simulink model "EstudioReguladores"  (R2024b)
settings: Solver=VariableStepAuto  StartTime=0.0  StopTime=50000  RelTol=1e-3
undefined symbols (not defined in the file): n, p1, p2, p3, Vi
libraries: slpidlib x32
(part 1 of 4)
settings Model: Creator=HP  LastModifiedBy=HP

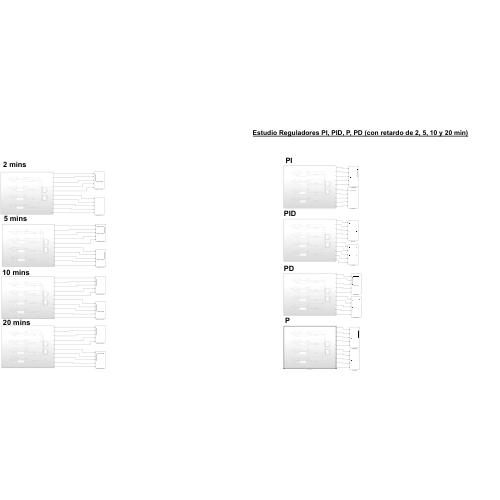
[thumbnail: Simulink's stored preview of the top-level diagram]
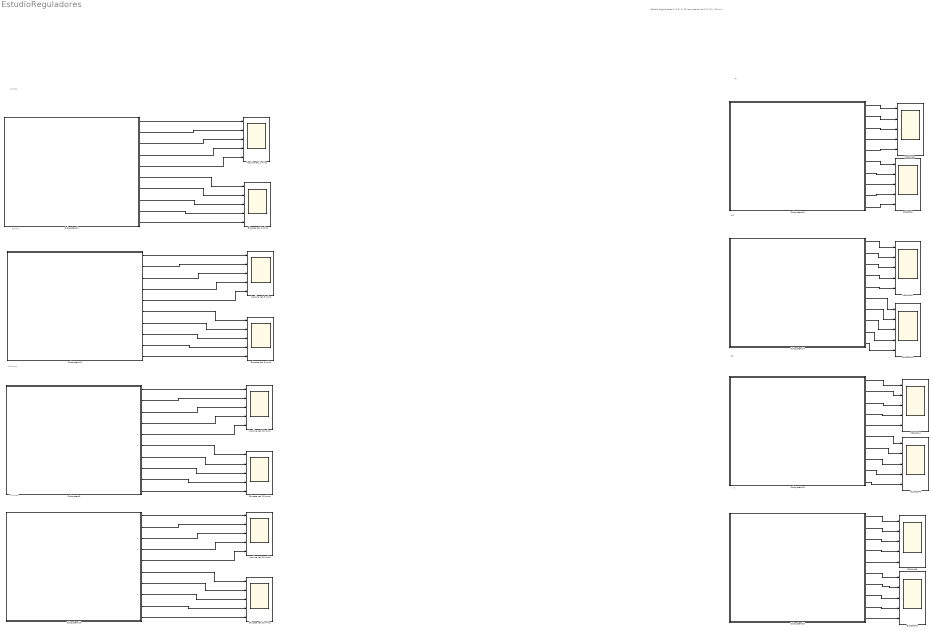
== system EstudioReguladores ==
  note: PI
  note: PID
  note: P
  note: 5 mins
  note: 2 mins
  note: Estudio Reguladores PI, PID, P, PD (con retardo de 2, 5, 10 y 20 min)
  note: 10 mins
  note: PD
  note: 20 mins
  GLUCOSA{,1..3} (4 alike) : Scope  NumInputPorts=5
  Glucosa ret. 10 mins. : Scope  NumInputPorts=5
  Glucosa ret. 2 mins : Scope  NumInputPorts=5
  Glucosa ret. 20 mins. : Scope  NumInputPorts=5
  Glucosa ret. 5 mins. : Scope  NumInputPorts=5
  INSULINA{2..5} (4 alike) : Scope  NumInputPorts=5
  Insulina ret. 10 mins. : Scope  NumInputPorts=5
  Insulina ret. 2 mins : Scope  NumInputPorts=5
  Insulina ret. 20 mins. : Scope  NumInputPorts=5
  Insulina ret. 5 mins. : Scope  NumInputPorts=5
  Subsystem10 : Subsystem
  Subsystem11 : Subsystem
  Subsystem12 : Subsystem
  Subsystem13 : Subsystem
  Subsystem14 : Subsystem
  Subsystem15 : Subsystem
  Subsystem16 : Subsystem
  Subsystem9 : Subsystem
  wires:
  Subsystem11/5(Out5) -> Insulina ret. 2 mins/5
  Subsystem16/7(Out7) -> GLUCOSA3/2
  Subsystem10/2(Out2) -> Insulina ret. 20 mins./2
  Subsystem11/3(Out3) -> Insulina ret. 2 mins/3
  Subsystem13/2(Out2) -> INSULINA2/2
  Subsystem13/10(Out10) -> GLUCOSA/5
  Subsystem10/4(Out4) -> Insulina ret. 20 mins./4
  Subsystem12/2(Out2) -> Insulina ret. 5 mins./2
  Subsystem13/1(Out1) -> INSULINA2/1
  Subsystem10/9(Out9) -> Glucosa ret. 20 mins./4
  Subsystem10/5(Out5) -> Insulina ret. 20 mins./5
  Subsystem10/1(Out1) -> Insulina ret. 20 mins./1
  Subsystem14/2(Out2) -> INSULINA3/2
  Subsystem12/4(Out4) -> Insulina ret. 5 mins./4
  Subsystem9/9(Out9) -> Glucosa ret. 10 mins./4
  Subsystem13/9(Out9) -> GLUCOSA/4
  Subsystem10/3(Out3) -> Insulina ret. 20 mins./3
  Subsystem14/7(Out7) -> GLUCOSA1/2
  Subsystem12/5(Out5) -> Insulina ret. 5 mins./5
  Subsystem12/1(Out1) -> Insulina ret. 5 mins./1
  Subsystem10/7(Out7) -> Glucosa ret. 20 mins./2
  Subsystem11/9(Out9) -> Glucosa ret. 2 mins/4
  Subsystem12/7(Out7) -> Glucosa ret. 5 mins./2
  Subsystem9/3(Out3) -> Insulina ret. 10 mins./3
  Subsystem11/1(Out1) -> Insulina ret. 2 mins/1
  Subsystem11/10(Out10) -> Glucosa ret. 2 mins/5
  Subsystem11/7(Out7) -> Glucosa ret. 2 mins/2
  Subsystem13/3(Out3) -> INSULINA2/3
  Subsystem16/6(Out6) -> GLUCOSA3/1
  Subsystem13/5(Out5) -> INSULINA2/5
  Subsystem15/8(Out8) -> GLUCOSA2/3
  Subsystem16/1(Out1) -> INSULINA5/1
  Subsystem13/4(Out4) -> INSULINA2/4
  Subsystem15/7(Out7) -> GLUCOSA2/2
  Subsystem9/5(Out5) -> Insulina ret. 10 mins./5
  Subsystem12/6(Out6) -> Glucosa ret. 5 mins./1
  Subsystem13/7(Out7) -> GLUCOSA/2
  Subsystem11/4(Out4) -> Insulina ret. 2 mins/4
  Subsystem9/10(Out10) -> Glucosa ret. 10 mins./5
  Subsystem12/9(Out9) -> Glucosa ret. 5 mins./4
  Subsystem9/1(Out1) -> Insulina ret. 10 mins./1
  Subsystem9/8(Out8) -> Glucosa ret. 10 mins./3
  Subsystem11/2(Out2) -> Insulina ret. 2 mins/2
  Subsystem9/7(Out7) -> Glucosa ret. 10 mins./2
  Subsystem13/6(Out6) -> GLUCOSA/1
  Subsystem12/10(Out10) -> Glucosa ret. 5 mins./5
  Subsystem11/6(Out6) -> Glucosa ret. 2 mins/1
  Subsystem13/8(Out8) -> GLUCOSA/3
  Subsystem9/4(Out4) -> Insulina ret. 10 mins./4
  Subsystem10/10(Out10) -> Glucosa ret. 20 mins./5
  Subsystem10/8(Out8) -> Glucosa ret. 20 mins./3
  Subsystem12/8(Out8) -> Glucosa ret. 5 mins./3
  Subsystem11/8(Out8) -> Glucosa ret. 2 mins/3
  Subsystem9/2(Out2) -> Insulina ret. 10 mins./2
  Subsystem10/6(Out6) -> Glucosa ret. 20 mins./1
  Subsystem12/3(Out3) -> Insulina ret. 5 mins./3
  Subsystem9/6(Out6) -> Glucosa ret. 10 mins./1
  Subsystem15/6(Out6) -> GLUCOSA2/1
  Subsystem14/6(Out6) -> GLUCOSA1/1
  Subsystem14/8(Out8) -> GLUCOSA1/3
  Subsystem14/9(Out9) -> GLUCOSA1/4
  Subsystem14/10(Out10) -> GLUCOSA1/5
  Subsystem14/1(Out1) -> INSULINA3/1
  Subsystem14/3(Out3) -> INSULINA3/3
  Subsystem14/4(Out4) -> INSULINA3/4
  Subsystem14/5(Out5) -> INSULINA3/5
  Subsystem15/1(Out1) -> INSULINA4/1
  Subsystem15/2(Out2) -> INSULINA4/2
  Subsystem15/3(Out3) -> INSULINA4/3
  Subsystem15/4(Out4) -> INSULINA4/4
  Subsystem15/5(Out5) -> INSULINA4/5
  Subsystem16/2(Out2) -> INSULINA5/2
  Subsystem16/3(Out3) -> INSULINA5/3
  Subsystem16/4(Out4) -> INSULINA5/4
  Subsystem16/5(Out5) -> INSULINA5/5
  Subsystem15/9(Out9) -> GLUCOSA2/4
  Subsystem15/10(Out10) -> GLUCOSA2/5
  Subsystem16/8(Out8) -> GLUCOSA3/3
  Subsystem16/9(Out9) -> GLUCOSA3/4
  Subsystem16/10(Out10) -> GLUCOSA3/5

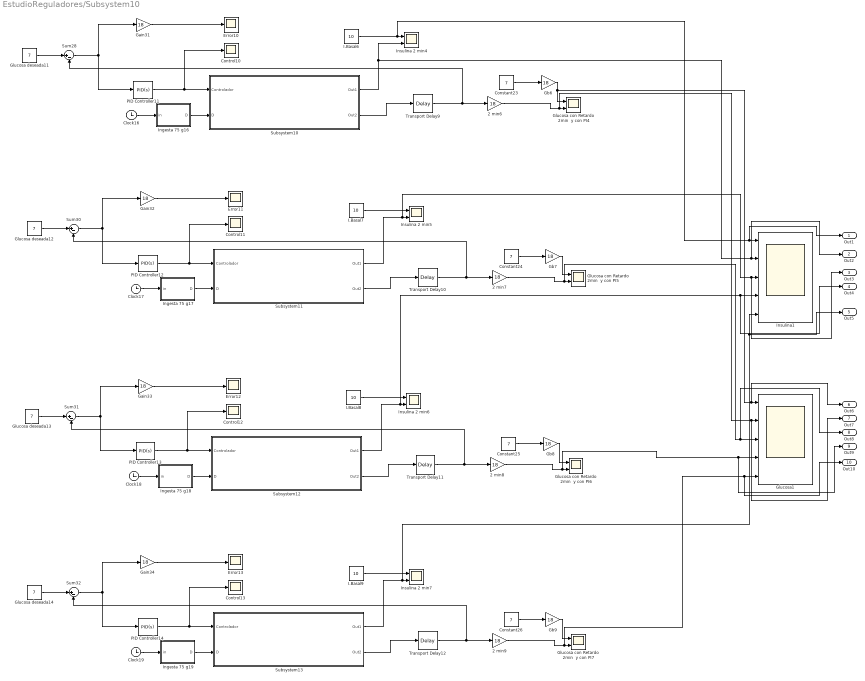
== system EstudioReguladores/Subsystem10 ==
  2 min{6..9} (4 alike) : Gain  Gain=18
  Clock{16..19} (4 alike) : Clock
  Constant{23..26} (4 alike) : Constant  Value=7
  Control{10..13} (4 alike) : Scope
  Error{10..13} (4 alike) : Scope
  Gain{31..34} (4 alike) : Gain  Gain=18
  Gb{6..9} (4 alike) : Gain  Gain=18
  Glucosa con Retardo 2min  y con PI{4..7} (4 alike) : Scope  NumInputPorts=2
  Glucosa deseada{11..14} (4 alike) : Constant  Value=7
  Glucosa1 : Scope  NumInputPorts=5
  I.Basal{6..9} (4 alike) : Constant  Value=10
  Ingesta 75 g16 : MATLAB Function  TreatAsAtomicUnit=on
  Ingesta 75 g17 : MATLAB Function  TreatAsAtomicUnit=on
  Ingesta 75 g18 : MATLAB Function  TreatAsAtomicUnit=on
  Ingesta 75 g19 : MATLAB Function  TreatAsAtomicUnit=on
  Insulina 2 min{4..7} (4 alike) : Scope  NumInputPorts=2
  Insulina1 : Scope  NumInputPorts=5
  PID Controller11 : slpidlib/PID Controller  Controller=PID  Form=Parallel  TimeDomain=Continuous-time  UseExternalTs=off  SampleTime=-1  IntegratorMethod=Forward Euler  FilterMethod=Forward Euler  ControllerParametersSource=internal  P=-0.3195  I=-0.3195/2998.95  UseKiTs=off  D=0  UseExternalDerivativeSource=off  N=10  UseFilter=on  TunerSelectOption=Transfer Function Based (PID Tuner App)  InitialConditionSource=internal  InitialConditionForIntegrator=0  InitialConditionForFilter=0  DifferentiatorICPrevScaledInput=0  ExternalReset=none  TrackingMode=off  Kt=1  LimitOutput=off  SatLimitsSource=internal  UpperSaturationLimit=inf  LowerSaturationLimit=-inf  LinearizeAsGain=on  AntiWindupMode=none  Kb=1  LimitIntegrator=off  UpperIntegratorSaturationLimit=inf  LowerIntegratorSaturationLimit=-inf  POutMin=[]  POutMax=[]  IOutMin=[]  IOutMax=[]  DOutMin=[]  DOutMax=[]  NOutMin=[]  NOutMax=[]  SumOutMin=[]  SumOutMax=[]  SaturationOutMin=[]  SaturationOutMax=[]  PParamMin=[]  PParamMax=[]  IParamMin=[]  IParamMax=[]  DParamMin=[]  DParamMax=[]  NParamMin=[]  NParamMax=[]  KbParamMin=[]  KbParamMax=[]  KtParamMin=[]  KtParamMax=[]  KbOutMin=[]  KbOutMax=[]  KtOutMin=[]  KtOutMax=[]  IntegratorOutMin=[]  IntegratorOutMax=[]  FilterOutMin=[]  FilterOutMax=[]  SumI1OutMin=[]  SumI1OutMax=[]  SumI2OutMin=[]  SumI2OutMax=[]  SumI3OutMin=[]  SumI3OutMax=[]  SumI4OutMin=[]  SumI4OutMax=[]  SumDOutMin=[]  SumDOutMax=[]  DifferentiatorOutMin=[]  DifferentiatorOutMax=[]  FilterDiffOutCoefMin=[]  FilterDiffOutCoefMax=[]  ReciprocalOutMin=[]  ReciprocalOutMax=[]  SumDenOutMin=[]  SumDenOutMax=[]  SumNumOutMin=[]  SumNumOutMax=[]  DivideOutMin=[]  DivideOutMax=[]  UdiffTsProdOutMin=[]  UdiffTsProdOutMax=[]  NTsProdOutMin=[]  NTsProdOutMax=[]  UintegralTsProdOutMin=[]  UintegralTsProdOutMax=[]  UngainTsProdOutMin=[]  UngainTsProdOutMax=[]  ClampingZeroOutDataTypeStr=Inherit: Inherit via back propagation  ClampingZeroOutMin=[]  ClampingZeroOutMax=[]  FilterDenConstantOutDataTypeStr=Inherit: Inherit via back propagation  FilterDenConstantOutMin=[]  FilterDenConstantOutMax=[]  PCopyOutDataTypeStr=Inherit: Inherit via back propagation  PCopyOutMin=[]  PCopyOutMax=[]  NCopyOutDataTypeStr=Inherit: Inherit via back propagation  NCopyOutMin=[]  NCopyOutMax=[]  IntegratorContinuousStateAttributes=''  IntegratorStateMustResolveToSignalObject=off  IntegratorRTWStateStorageClass=Auto  FilterContinuousStateAttributes=''  FilterStateMustResolveToSignalObject=off  FilterRTWStateStorageClass=Auto  ParallelPVariant=InternalParameters  IdealPVariant=Disabled  IVariant=InternalParameters  DVariant=InternalParameters  IntegratorVariant=Continuous  SatVariant=Disabled  AWVariant=Passthrough  PCopyVariant=Disabled  TRVariant=Disabled  FdbkBlocksVariant=Forward  IdealPFdbkVariant=Disabled  SatFdbkVariant=Disabled  DerivativeFilterVariant=ContFilter  NVariant=InternalParameters  NCopyVariant=Disabled  FilterICVariant=InternalICsFilter  IntegratorICVariant=InternalICs  ExternalResetVariant=Disabled  TRSumVariant=Passthrough  SumFdbkVariant=Disabled  SumVariant=Sum_PID  TsampFilterVariant=InternalTs  TsampNgainVariant=Passthrough  TsampIntegralVariant=Disabled_SignalSpec  ExternalSaturationOutDataTypeStr=Inherit: Same as second input  DerivativeSourceVariant=ErrorSignal  PreIntVariant=InternalPreInt
  PID Controller12 : slpidlib/PID Controller  Controller=PID  Form=Parallel  TimeDomain=Continuous-time  UseExternalTs=off  SampleTime=-1  IntegratorMethod=Forward Euler  FilterMethod=Forward Euler  ControllerParametersSource=internal  P=-0.3195  I=-0.3195/2998.95  UseKiTs=off  D=0.01  UseExternalDerivativeSource=off  N=10  UseFilter=on  TunerSelectOption=Transfer Function Based (PID Tuner App)  InitialConditionSource=internal  InitialConditionForIntegrator=0  InitialConditionForFilter=0  DifferentiatorICPrevScaledInput=0  ExternalReset=none  TrackingMode=off  Kt=1  LimitOutput=off  SatLimitsSource=internal  UpperSaturationLimit=inf  LowerSaturationLimit=-inf  LinearizeAsGain=on  AntiWindupMode=none  Kb=1  LimitIntegrator=off  UpperIntegratorSaturationLimit=inf  LowerIntegratorSaturationLimit=-inf  POutMin=[]  POutMax=[]  IOutMin=[]  IOutMax=[]  DOutMin=[]  DOutMax=[]  NOutMin=[]  NOutMax=[]  SumOutMin=[]  SumOutMax=[]  SaturationOutMin=[]  SaturationOutMax=[]  PParamMin=[]  PParamMax=[]  IParamMin=[]  IParamMax=[]  DParamMin=[]  DParamMax=[]  NParamMin=[]  NParamMax=[]  KbParamMin=[]  KbParamMax=[]  KtParamMin=[]  KtParamMax=[]  KbOutMin=[]  KbOutMax=[]  KtOutMin=[]  KtOutMax=[]  IntegratorOutMin=[]  IntegratorOutMax=[]  FilterOutMin=[]  FilterOutMax=[]  SumI1OutMin=[]  SumI1OutMax=[]  SumI2OutMin=[]  SumI2OutMax=[]  SumI3OutMin=[]  SumI3OutMax=[]  SumI4OutMin=[]  SumI4OutMax=[]  SumDOutMin=[]  SumDOutMax=[]  DifferentiatorOutMin=[]  DifferentiatorOutMax=[]  FilterDiffOutCoefMin=[]  FilterDiffOutCoefMax=[]  ReciprocalOutMin=[]  ReciprocalOutMax=[]  SumDenOutMin=[]  SumDenOutMax=[]  SumNumOutMin=[]  SumNumOutMax=[]  DivideOutMin=[]  DivideOutMax=[]  UdiffTsProdOutMin=[]  UdiffTsProdOutMax=[]  NTsProdOutMin=[]  NTsProdOutMax=[]  UintegralTsProdOutMin=[]  UintegralTsProdOutMax=[]  UngainTsProdOutMin=[]  UngainTsProdOutMax=[]  ClampingZeroOutDataTypeStr=Inherit: Inherit via back propagation  ClampingZeroOutMin=[]  ClampingZeroOutMax=[]  FilterDenConstantOutDataTypeStr=Inherit: Inherit via back propagation  FilterDenConstantOutMin=[]  FilterDenConstantOutMax=[]  PCopyOutDataTypeStr=Inherit: Inherit via back propagation  PCopyOutMin=[]  PCopyOutMax=[]  NCopyOutDataTypeStr=Inherit: Inherit via back propagation  NCopyOutMin=[]  NCopyOutMax=[]  IntegratorContinuousStateAttributes=''  IntegratorStateMustResolveToSignalObject=off  IntegratorRTWStateStorageClass=Auto  FilterContinuousStateAttributes=''  FilterStateMustResolveToSignalObject=off  FilterRTWStateStorageClass=Auto  ParallelPVariant=InternalParameters  IdealPVariant=Disabled  IVariant=InternalParameters  DVariant=InternalParameters  IntegratorVariant=Continuous  SatVariant=Disabled  AWVariant=Passthrough  PCopyVariant=Disabled  TRVariant=Disabled  FdbkBlocksVariant=Forward  IdealPFdbkVariant=Disabled  SatFdbkVariant=Disabled  DerivativeFilterVariant=ContFilter  NVariant=InternalParameters  NCopyVariant=Disabled  FilterICVariant=InternalICsFilter  IntegratorICVariant=InternalICs  ExternalResetVariant=Disabled  TRSumVariant=Passthrough  SumFdbkVariant=Disabled  SumVariant=Sum_PID  TsampFilterVariant=InternalTs  TsampNgainVariant=Passthrough  TsampIntegralVariant=Disabled_SignalSpec  ExternalSaturationOutDataTypeStr=Inherit: Same as second input  DerivativeSourceVariant=ErrorSignal  PreIntVariant=InternalPreInt
  PID Controller13 : slpidlib/PID Controller  Controller=PID  Form=Parallel  TimeDomain=Continuous-time  UseExternalTs=off  SampleTime=-1  IntegratorMethod=Forward Euler  FilterMethod=Forward Euler  ControllerParametersSource=internal  P=-0.3195  I=0  UseKiTs=off  D=0  UseExternalDerivativeSource=off  N=10  UseFilter=on  TunerSelectOption=Transfer Function Based (PID Tuner App)  InitialConditionSource=internal  InitialConditionForIntegrator=0  InitialConditionForFilter=0  DifferentiatorICPrevScaledInput=0  ExternalReset=none  TrackingMode=off  Kt=1  LimitOutput=off  SatLimitsSource=internal  UpperSaturationLimit=inf  LowerSaturationLimit=-inf  LinearizeAsGain=on  AntiWindupMode=none  Kb=1  LimitIntegrator=off  UpperIntegratorSaturationLimit=inf  LowerIntegratorSaturationLimit=-inf  POutMin=[]  POutMax=[]  IOutMin=[]  IOutMax=[]  DOutMin=[]  DOutMax=[]  NOutMin=[]  NOutMax=[]  SumOutMin=[]  SumOutMax=[]  SaturationOutMin=[]  SaturationOutMax=[]  PParamMin=[]  PParamMax=[]  IParamMin=[]  IParamMax=[]  DParamMin=[]  DParamMax=[]  NParamMin=[]  NParamMax=[]  KbParamMin=[]  KbParamMax=[]  KtParamMin=[]  KtParamMax=[]  KbOutMin=[]  KbOutMax=[]  KtOutMin=[]  KtOutMax=[]  IntegratorOutMin=[]  IntegratorOutMax=[]  FilterOutMin=[]  FilterOutMax=[]  SumI1OutMin=[]  SumI1OutMax=[]  SumI2OutMin=[]  SumI2OutMax=[]  SumI3OutMin=[]  SumI3OutMax=[]  SumI4OutMin=[]  SumI4OutMax=[]  SumDOutMin=[]  SumDOutMax=[]  DifferentiatorOutMin=[]  DifferentiatorOutMax=[]  FilterDiffOutCoefMin=[]  FilterDiffOutCoefMax=[]  ReciprocalOutMin=[]  ReciprocalOutMax=[]  SumDenOutMin=[]  SumDenOutMax=[]  SumNumOutMin=[]  SumNumOutMax=[]  DivideOutMin=[]  DivideOutMax=[]  UdiffTsProdOutMin=[]  UdiffTsProdOutMax=[]  NTsProdOutMin=[]  NTsProdOutMax=[]  UintegralTsProdOutMin=[]  UintegralTsProdOutMax=[]  UngainTsProdOutMin=[]  UngainTsProdOutMax=[]  ClampingZeroOutDataTypeStr=Inherit: Inherit via back propagation  ClampingZeroOutMin=[]  ClampingZeroOutMax=[]  FilterDenConstantOutDataTypeStr=Inherit: Inherit via back propagation  FilterDenConstantOutMin=[]  FilterDenConstantOutMax=[]  PCopyOutDataTypeStr=Inherit: Inherit via back propagation  PCopyOutMin=[]  PCopyOutMax=[]  NCopyOutDataTypeStr=Inherit: Inherit via back propagation  NCopyOutMin=[]  NCopyOutMax=[]  IntegratorContinuousStateAttributes=''  IntegratorStateMustResolveToSignalObject=off  IntegratorRTWStateStorageClass=Auto  FilterContinuousStateAttributes=''  FilterStateMustResolveToSignalObject=off  FilterRTWStateStorageClass=Auto  ParallelPVariant=InternalParameters  IdealPVariant=Disabled  IVariant=InternalParameters  DVariant=InternalParameters  IntegratorVariant=Continuous  SatVariant=Disabled  AWVariant=Passthrough  PCopyVariant=Disabled  TRVariant=Disabled  FdbkBlocksVariant=Forward  IdealPFdbkVariant=Disabled  SatFdbkVariant=Disabled  DerivativeFilterVariant=ContFilter  NVariant=InternalParameters  NCopyVariant=Disabled  FilterICVariant=InternalICsFilter  IntegratorICVariant=InternalICs  ExternalResetVariant=Disabled  TRSumVariant=Passthrough  SumFdbkVariant=Disabled  SumVariant=Sum_PID  TsampFilterVariant=InternalTs  TsampNgainVariant=Passthrough  TsampIntegralVariant=Disabled_SignalSpec  ExternalSaturationOutDataTypeStr=Inherit: Same as second input  DerivativeSourceVariant=ErrorSignal  PreIntVariant=InternalPreInt
  PID Controller14 : slpidlib/PID Controller  Controller=PID  Form=Parallel  TimeDomain=Continuous-time  UseExternalTs=off  SampleTime=-1  IntegratorMethod=Forward Euler  FilterMethod=Forward Euler  ControllerParametersSource=internal  P=-0.3195  I=0  UseKiTs=off  D=0.01  UseExternalDerivativeSource=off  N=10  UseFilter=on  TunerSelectOption=Transfer Function Based (PID Tuner App)  InitialConditionSource=internal  InitialConditionForIntegrator=0  InitialConditionForFilter=0  DifferentiatorICPrevScaledInput=0  ExternalReset=none  TrackingMode=off  Kt=1  LimitOutput=off  SatLimitsSource=internal  UpperSaturationLimit=inf  LowerSaturationLimit=-inf  LinearizeAsGain=on  AntiWindupMode=none  Kb=1  LimitIntegrator=off  UpperIntegratorSaturationLimit=inf  LowerIntegratorSaturationLimit=-inf  POutMin=[]  POutMax=[]  IOutMin=[]  IOutMax=[]  DOutMin=[]  DOutMax=[]  NOutMin=[]  NOutMax=[]  SumOutMin=[]  SumOutMax=[]  SaturationOutMin=[]  SaturationOutMax=[]  PParamMin=[]  PParamMax=[]  IParamMin=[]  IParamMax=[]  DParamMin=[]  DParamMax=[]  NParamMin=[]  NParamMax=[]  KbParamMin=[]  KbParamMax=[]  KtParamMin=[]  KtParamMax=[]  KbOutMin=[]  KbOutMax=[]  KtOutMin=[]  KtOutMax=[]  IntegratorOutMin=[]  IntegratorOutMax=[]  FilterOutMin=[]  FilterOutMax=[]  SumI1OutMin=[]  SumI1OutMax=[]  SumI2OutMin=[]  SumI2OutMax=[]  SumI3OutMin=[]  SumI3OutMax=[]  SumI4OutMin=[]  SumI4OutMax=[]  SumDOutMin=[]  SumDOutMax=[]  DifferentiatorOutMin=[]  DifferentiatorOutMax=[]  FilterDiffOutCoefMin=[]  FilterDiffOutCoefMax=[]  ReciprocalOutMin=[]  ReciprocalOutMax=[]  SumDenOutMin=[]  SumDenOutMax=[]  SumNumOutMin=[]  SumNumOutMax=[]  DivideOutMin=[]  DivideOutMax=[]  UdiffTsProdOutMin=[]  UdiffTsProdOutMax=[]  NTsProdOutMin=[]  NTsProdOutMax=[]  UintegralTsProdOutMin=[]  UintegralTsProdOutMax=[]  UngainTsProdOutMin=[]  UngainTsProdOutMax=[]  ClampingZeroOutDataTypeStr=Inherit: Inherit via back propagation  ClampingZeroOutMin=[]  ClampingZeroOutMax=[]  FilterDenConstantOutDataTypeStr=Inherit: Inherit via back propagation  FilterDenConstantOutMin=[]  FilterDenConstantOutMax=[]  PCopyOutDataTypeStr=Inherit: Inherit via back propagation  PCopyOutMin=[]  PCopyOutMax=[]  NCopyOutDataTypeStr=Inherit: Inherit via back propagation  NCopyOutMin=[]  NCopyOutMax=[]  IntegratorContinuousStateAttributes=''  IntegratorStateMustResolveToSignalObject=off  IntegratorRTWStateStorageClass=Auto  FilterContinuousStateAttributes=''  FilterStateMustResolveToSignalObject=off  FilterRTWStateStorageClass=Auto  ParallelPVariant=InternalParameters  IdealPVariant=Disabled  IVariant=InternalParameters  DVariant=InternalParameters  IntegratorVariant=Continuous  SatVariant=Disabled  AWVariant=Passthrough  PCopyVariant=Disabled  TRVariant=Disabled  FdbkBlocksVariant=Forward  IdealPFdbkVariant=Disabled  SatFdbkVariant=Disabled  DerivativeFilterVariant=ContFilter  NVariant=InternalParameters  NCopyVariant=Disabled  FilterICVariant=InternalICsFilter  IntegratorICVariant=InternalICs  ExternalResetVariant=Disabled  TRSumVariant=Passthrough  SumFdbkVariant=Disabled  SumVariant=Sum_PID  TsampFilterVariant=InternalTs  TsampNgainVariant=Passthrough  TsampIntegralVariant=Disabled_SignalSpec  ExternalSaturationOutDataTypeStr=Inherit: Same as second input  DerivativeSourceVariant=ErrorSignal  PreIntVariant=InternalPreInt
  Subsystem10 : Subsystem
  Subsystem11 : Subsystem
  Subsystem12 : Subsystem
  Subsystem13 : Subsystem
  Sum{28,30..32} (4 alike) : Sum  Inputs=|+-
  Transport Delay{9..12} (4 alike) : TransportDelay  DelayTime=1200  InitialOutput=7
  Out1 : Outport
  Out2 : Outport  Port=2
  Out3 : Outport  Port=3
  Out4 : Outport  Port=4
  Out5 : Outport  Port=5
  Out6 : Outport  Port=6
  Out7 : Outport  Port=7
  Out8 : Outport  Port=8
  Out9 : Outport  Port=9
  Out10 : Outport  Port=10
  wires:
  Glucosa deseada13/1 -> Sum31/1
  Subsystem12/1(Out1) -> Out4/1, Insulina1/4, Insulina 2 min6/2
  2 min9/1 -> Out10/1, Glucosa1/5, Glucosa con Retardo 2min  y con PI7/2
  I.Basal6/1 -> Out1/1, Insulina1/1, Insulina 2 min4/1
  Transport Delay12/1 -> Sum32/2, 2 min9/1
  Glucosa deseada14/1 -> Sum32/1
  Gain31/1 -> Error10/1
  I.Basal9/1 -> Insulina 2 min7/1
  PID Controller13/1 -> Control12/1, Subsystem12/1(Controlador)
  Glucosa deseada11/1 -> Sum28/1
  I.Basal8/1 -> Insulina 2 min6/1
  Ingesta 75 g19/1(D) -> Subsystem13/2(D)
  Gb8/1 -> Glucosa con Retardo 2min  y con PI6/1
  2 min8/1 -> Out9/1, Glucosa1/4, Glucosa con Retardo 2min  y con PI6/2
  PID Controller12/1 -> Control11/1, Subsystem11/1(Controlador)
  Gb9/1 -> Glucosa con Retardo 2min  y con PI7/1
  Sum32/1 -> PID Controller14/1, Gain34/1
  Gb6/1 -> Out6/1, Glucosa1/1, Glucosa con Retardo 2min  y con PI4/1
  Transport Delay11/1 -> Sum31/2, 2 min8/1
  Clock18/1 -> Ingesta 75 g18/1(in)
  PID Controller14/1 -> Control13/1, Subsystem13/1(Controlador)
  Subsystem10/1(Out1) -> Insulina 2 min4/2, Out2/1, Insulina1/2
  PID Controller11/1 -> Control10/1, Subsystem10/1(Controlador)
  2 min6/1 -> Out7/1, Glucosa1/2, Glucosa con Retardo 2min  y con PI4/2
  Subsystem12/2(Out2) -> Transport Delay11/1
  Gb7/1 -> Glucosa con Retardo 2min  y con PI5/1
  Subsystem13/1(Out1) -> Out5/1, Insulina1/5, Insulina 2 min7/2
  Sum31/1 -> PID Controller13/1, Gain33/1
  2 min7/1 -> Out8/1, Glucosa1/3, Glucosa con Retardo 2min  y con PI5/2
  Subsystem13/2(Out2) -> Transport Delay12/1
  Gain33/1 -> Error12/1
  Transport Delay9/1 -> Sum28/2, 2 min6/1
  Constant25/1 -> Gb8/1
  Ingesta 75 g17/1(D) -> Subsystem11/2(D)
  Ingesta 75 g18/1(D) -> Subsystem12/2(D)
  Gain34/1 -> Error13/1
  Clock19/1 -> Ingesta 75 g19/1(in)
  Glucosa deseada12/1 -> Sum30/1
  Constant26/1 -> Gb9/1
  Ingesta 75 g16/1(D) -> Subsystem10/2(D)
  Subsystem11/1(Out1) -> Out3/1, Insulina1/3, Insulina 2 min5/2
  Sum28/1 -> PID Controller11/1, Gain31/1
  Constant23/1 -> Gb6/1
  Sum30/1 -> PID Controller12/1, Gain32/1
  Transport Delay10/1 -> Sum30/2, 2 min7/1
  I.Basal7/1 -> Insulina 2 min5/1
  Subsystem11/2(Out2) -> Transport Delay10/1
  Clock17/1 -> Ingesta 75 g17/1(in)
  Subsystem10/2(Out2) -> Transport Delay9/1
  Constant24/1 -> Gb7/1
  Gain32/1 -> Error11/1
  Clock16/1 -> Ingesta 75 g16/1(in)

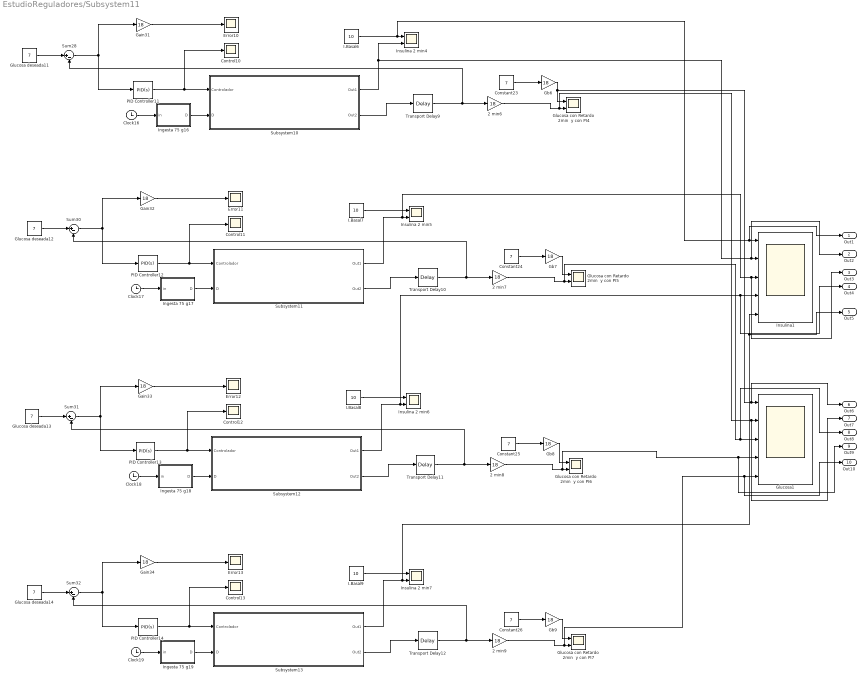
== system EstudioReguladores/Subsystem11 ==
  2 min{6..9} (4 alike) : Gain  Gain=18
  Clock{16..19} (4 alike) : Clock
  Constant{23..26} (4 alike) : Constant  Value=7
  Control{10..13} (4 alike) : Scope
  Error{10..13} (4 alike) : Scope
  Gain{31..34} (4 alike) : Gain  Gain=18
  Gb{6..9} (4 alike) : Gain  Gain=18
  Glucosa con Retardo 2min  y con PI{4..7} (4 alike) : Scope  NumInputPorts=2
  Glucosa deseada{11..14} (4 alike) : Constant  Value=7
  Glucosa1 : Scope  NumInputPorts=5
  I.Basal{6..9} (4 alike) : Constant  Value=10
  Ingesta 75 g16 : MATLAB Function  TreatAsAtomicUnit=on
  Ingesta 75 g17 : MATLAB Function  TreatAsAtomicUnit=on
  Ingesta 75 g18 : MATLAB Function  TreatAsAtomicUnit=on
  Ingesta 75 g19 : MATLAB Function  TreatAsAtomicUnit=on
  Insulina 2 min{4..7} (4 alike) : Scope  NumInputPorts=2
  Insulina1 : Scope  NumInputPorts=5
  PID Controller11 : slpidlib/PID Controller  Controller=PID  Form=Parallel  TimeDomain=Continuous-time  UseExternalTs=off  SampleTime=-1  IntegratorMethod=Forward Euler  FilterMethod=Forward Euler  ControllerParametersSource=internal  P=-0.3195  I=-0.3195/2998.95  UseKiTs=off  D=0  UseExternalDerivativeSource=off  N=10  UseFilter=on  TunerSelectOption=Transfer Function Based (PID Tuner App)  InitialConditionSource=internal  InitialConditionForIntegrator=0  InitialConditionForFilter=0  DifferentiatorICPrevScaledInput=0  ExternalReset=none  TrackingMode=off  Kt=1  LimitOutput=off  SatLimitsSource=internal  UpperSaturationLimit=inf  LowerSaturationLimit=-inf  LinearizeAsGain=on  AntiWindupMode=none  Kb=1  LimitIntegrator=off  UpperIntegratorSaturationLimit=inf  LowerIntegratorSaturationLimit=-inf  POutMin=[]  POutMax=[]  IOutMin=[]  IOutMax=[]  DOutMin=[]  DOutMax=[]  NOutMin=[]  NOutMax=[]  SumOutMin=[]  SumOutMax=[]  SaturationOutMin=[]  SaturationOutMax=[]  PParamMin=[]  PParamMax=[]  IParamMin=[]  IParamMax=[]  DParamMin=[]  DParamMax=[]  NParamMin=[]  NParamMax=[]  KbParamMin=[]  KbParamMax=[]  KtParamMin=[]  KtParamMax=[]  KbOutMin=[]  KbOutMax=[]  KtOutMin=[]  KtOutMax=[]  IntegratorOutMin=[]  IntegratorOutMax=[]  FilterOutMin=[]  FilterOutMax=[]  SumI1OutMin=[]  SumI1OutMax=[]  SumI2OutMin=[]  SumI2OutMax=[]  SumI3OutMin=[]  SumI3OutMax=[]  SumI4OutMin=[]  SumI4OutMax=[]  SumDOutMin=[]  SumDOutMax=[]  DifferentiatorOutMin=[]  DifferentiatorOutMax=[]  FilterDiffOutCoefMin=[]  FilterDiffOutCoefMax=[]  ReciprocalOutMin=[]  ReciprocalOutMax=[]  SumDenOutMin=[]  SumDenOutMax=[]  SumNumOutMin=[]  SumNumOutMax=[]  DivideOutMin=[]  DivideOutMax=[]  UdiffTsProdOutMin=[]  UdiffTsProdOutMax=[]  NTsProdOutMin=[]  NTsProdOutMax=[]  UintegralTsProdOutMin=[]  UintegralTsProdOutMax=[]  UngainTsProdOutMin=[]  UngainTsProdOutMax=[]  ClampingZeroOutDataTypeStr=Inherit: Inherit via back propagation  ClampingZeroOutMin=[]  ClampingZeroOutMax=[]  FilterDenConstantOutDataTypeStr=Inherit: Inherit via back propagation  FilterDenConstantOutMin=[]  FilterDenConstantOutMax=[]  PCopyOutDataTypeStr=Inherit: Inherit via back propagation  PCopyOutMin=[]  PCopyOutMax=[]  NCopyOutDataTypeStr=Inherit: Inherit via back propagation  NCopyOutMin=[]  NCopyOutMax=[]  IntegratorContinuousStateAttributes=''  IntegratorStateMustResolveToSignalObject=off  IntegratorRTWStateStorageClass=Auto  FilterContinuousStateAttributes=''  FilterStateMustResolveToSignalObject=off  FilterRTWStateStorageClass=Auto  ParallelPVariant=InternalParameters  IdealPVariant=Disabled  IVariant=InternalParameters  DVariant=InternalParameters  IntegratorVariant=Continuous  SatVariant=Disabled  AWVariant=Passthrough  PCopyVariant=Disabled  TRVariant=Disabled  FdbkBlocksVariant=Forward  IdealPFdbkVariant=Disabled  SatFdbkVariant=Disabled  DerivativeFilterVariant=ContFilter  NVariant=InternalParameters  NCopyVariant=Disabled  FilterICVariant=InternalICsFilter  IntegratorICVariant=InternalICs  ExternalResetVariant=Disabled  TRSumVariant=Passthrough  SumFdbkVariant=Disabled  SumVariant=Sum_PID  TsampFilterVariant=InternalTs  TsampNgainVariant=Passthrough  TsampIntegralVariant=Disabled_SignalSpec  ExternalSaturationOutDataTypeStr=Inherit: Same as second input  DerivativeSourceVariant=ErrorSignal  PreIntVariant=InternalPreInt
  PID Controller12 : slpidlib/PID Controller  Controller=PID  Form=Parallel  TimeDomain=Continuous-time  UseExternalTs=off  SampleTime=-1  IntegratorMethod=Forward Euler  FilterMethod=Forward Euler  ControllerParametersSource=internal  P=-0.3195  I=-0.3195/2998.95  UseKiTs=off  D=0.01  UseExternalDerivativeSource=off  N=10  UseFilter=on  TunerSelectOption=Transfer Function Based (PID Tuner App)  InitialConditionSource=internal  InitialConditionForIntegrator=0  InitialConditionForFilter=0  DifferentiatorICPrevScaledInput=0  ExternalReset=none  TrackingMode=off  Kt=1  LimitOutput=off  SatLimitsSource=internal  UpperSaturationLimit=inf  LowerSaturationLimit=-inf  LinearizeAsGain=on  AntiWindupMode=none  Kb=1  LimitIntegrator=off  UpperIntegratorSaturationLimit=inf  LowerIntegratorSaturationLimit=-inf  POutMin=[]  POutMax=[]  IOutMin=[]  IOutMax=[]  DOutMin=[]  DOutMax=[]  NOutMin=[]  NOutMax=[]  SumOutMin=[]  SumOutMax=[]  SaturationOutMin=[]  SaturationOutMax=[]  PParamMin=[]  PParamMax=[]  IParamMin=[]  IParamMax=[]  DParamMin=[]  DParamMax=[]  NParamMin=[]  NParamMax=[]  KbParamMin=[]  KbParamMax=[]  KtParamMin=[]  KtParamMax=[]  KbOutMin=[]  KbOutMax=[]  KtOutMin=[]  KtOutMax=[]  IntegratorOutMin=[]  IntegratorOutMax=[]  FilterOutMin=[]  FilterOutMax=[]  SumI1OutMin=[]  SumI1OutMax=[]  SumI2OutMin=[]  SumI2OutMax=[]  SumI3OutMin=[]  SumI3OutMax=[]  SumI4OutMin=[]  SumI4OutMax=[]  SumDOutMin=[]  SumDOutMax=[]  DifferentiatorOutMin=[]  DifferentiatorOutMax=[]  FilterDiffOutCoefMin=[]  FilterDiffOutCoefMax=[]  ReciprocalOutMin=[]  ReciprocalOutMax=[]  SumDenOutMin=[]  SumDenOutMax=[]  SumNumOutMin=[]  SumNumOutMax=[]  DivideOutMin=[]  DivideOutMax=[]  UdiffTsProdOutMin=[]  UdiffTsProdOutMax=[]  NTsProdOutMin=[]  NTsProdOutMax=[]  UintegralTsProdOutMin=[]  UintegralTsProdOutMax=[]  UngainTsProdOutMin=[]  UngainTsProdOutMax=[]  ClampingZeroOutDataTypeStr=Inherit: Inherit via back propagation  ClampingZeroOutMin=[]  ClampingZeroOutMax=[]  FilterDenConstantOutDataTypeStr=Inherit: Inherit via back propagation  FilterDenConstantOutMin=[]  FilterDenConstantOutMax=[]  PCopyOutDataTypeStr=Inherit: Inherit via back propagation  PCopyOutMin=[]  PCopyOutMax=[]  NCopyOutDataTypeStr=Inherit: Inherit via back propagation  NCopyOutMin=[]  NCopyOutMax=[]  IntegratorContinuousStateAttributes=''  IntegratorStateMustResolveToSignalObject=off  IntegratorRTWStateStorageClass=Auto  FilterContinuousStateAttributes=''  FilterStateMustResolveToSignalObject=off  FilterRTWStateStorageClass=Auto  ParallelPVariant=InternalParameters  IdealPVariant=Disabled  IVariant=InternalParameters  DVariant=InternalParameters  IntegratorVariant=Continuous  SatVariant=Disabled  AWVariant=Passthrough  PCopyVariant=Disabled  TRVariant=Disabled  FdbkBlocksVariant=Forward  IdealPFdbkVariant=Disabled  SatFdbkVariant=Disabled  DerivativeFilterVariant=ContFilter  NVariant=InternalParameters  NCopyVariant=Disabled  FilterICVariant=InternalICsFilter  IntegratorICVariant=InternalICs  ExternalResetVariant=Disabled  TRSumVariant=Passthrough  SumFdbkVariant=Disabled  SumVariant=Sum_PID  TsampFilterVariant=InternalTs  TsampNgainVariant=Passthrough  TsampIntegralVariant=Disabled_SignalSpec  ExternalSaturationOutDataTypeStr=Inherit: Same as second input  DerivativeSourceVariant=ErrorSignal  PreIntVariant=InternalPreInt
  PID Controller13 : slpidlib/PID Controller  Controller=PID  Form=Parallel  TimeDomain=Continuous-time  UseExternalTs=off  SampleTime=-1  IntegratorMethod=Forward Euler  FilterMethod=Forward Euler  ControllerParametersSource=internal  P=-0.3195  I=0  UseKiTs=off  D=0  UseExternalDerivativeSource=off  N=10  UseFilter=on  TunerSelectOption=Transfer Function Based (PID Tuner App)  InitialConditionSource=internal  InitialConditionForIntegrator=0  InitialConditionForFilter=0  DifferentiatorICPrevScaledInput=0  ExternalReset=none  TrackingMode=off  Kt=1  LimitOutput=off  SatLimitsSource=internal  UpperSaturationLimit=inf  LowerSaturationLimit=-inf  LinearizeAsGain=on  AntiWindupMode=none  Kb=1  LimitIntegrator=off  UpperIntegratorSaturationLimit=inf  LowerIntegratorSaturationLimit=-inf  POutMin=[]  POutMax=[]  IOutMin=[]  IOutMax=[]  DOutMin=[]  DOutMax=[]  NOutMin=[]  NOutMax=[]  SumOutMin=[]  SumOutMax=[]  SaturationOutMin=[]  SaturationOutMax=[]  PParamMin=[]  PParamMax=[]  IParamMin=[]  IParamMax=[]  DParamMin=[]  DParamMax=[]  NParamMin=[]  NParamMax=[]  KbParamMin=[]  KbParamMax=[]  KtParamMin=[]  KtParamMax=[]  KbOutMin=[]  KbOutMax=[]  KtOutMin=[]  KtOutMax=[]  IntegratorOutMin=[]  IntegratorOutMax=[]  FilterOutMin=[]  FilterOutMax=[]  SumI1OutMin=[]  SumI1OutMax=[]  SumI2OutMin=[]  SumI2OutMax=[]  SumI3OutMin=[]  SumI3OutMax=[]  SumI4OutMin=[]  SumI4OutMax=[]  SumDOutMin=[]  SumDOutMax=[]  DifferentiatorOutMin=[]  DifferentiatorOutMax=[]  FilterDiffOutCoefMin=[]  FilterDiffOutCoefMax=[]  ReciprocalOutMin=[]  ReciprocalOutMax=[]  SumDenOutMin=[]  SumDenOutMax=[]  SumNumOutMin=[]  SumNumOutMax=[]  DivideOutMin=[]  DivideOutMax=[]  UdiffTsProdOutMin=[]  UdiffTsProdOutMax=[]  NTsProdOutMin=[]  NTsProdOutMax=[]  UintegralTsProdOutMin=[]  UintegralTsProdOutMax=[]  UngainTsProdOutMin=[]  UngainTsProdOutMax=[]  ClampingZeroOutDataTypeStr=Inherit: Inherit via back propagation  ClampingZeroOutMin=[]  ClampingZeroOutMax=[]  FilterDenConstantOutDataTypeStr=Inherit: Inherit via back propagation  FilterDenConstantOutMin=[]  FilterDenConstantOutMax=[]  PCopyOutDataTypeStr=Inherit: Inherit via back propagation  PCopyOutMin=[]  PCopyOutMax=[]  NCopyOutDataTypeStr=Inherit: Inherit via back propagation  NCopyOutMin=[]  NCopyOutMax=[]  IntegratorContinuousStateAttributes=''  IntegratorStateMustResolveToSignalObject=off  IntegratorRTWStateStorageClass=Auto  FilterContinuousStateAttributes=''  FilterStateMustResolveToSignalObject=off  FilterRTWStateStorageClass=Auto  ParallelPVariant=InternalParameters  IdealPVariant=Disabled  IVariant=InternalParameters  DVariant=InternalParameters  IntegratorVariant=Continuous  SatVariant=Disabled  AWVariant=Passthrough  PCopyVariant=Disabled  TRVariant=Disabled  FdbkBlocksVariant=Forward  IdealPFdbkVariant=Disabled  SatFdbkVariant=Disabled  DerivativeFilterVariant=ContFilter  NVariant=InternalParameters  NCopyVariant=Disabled  FilterICVariant=InternalICsFilter  IntegratorICVariant=InternalICs  ExternalResetVariant=Disabled  TRSumVariant=Passthrough  SumFdbkVariant=Disabled  SumVariant=Sum_PID  TsampFilterVariant=InternalTs  TsampNgainVariant=Passthrough  TsampIntegralVariant=Disabled_SignalSpec  ExternalSaturationOutDataTypeStr=Inherit: Same as second input  DerivativeSourceVariant=ErrorSignal  PreIntVariant=InternalPreInt
  PID Controller14 : slpidlib/PID Controller  Controller=PID  Form=Parallel  TimeDomain=Continuous-time  UseExternalTs=off  SampleTime=-1  IntegratorMethod=Forward Euler  FilterMethod=Forward Euler  ControllerParametersSource=internal  P=-0.3195  I=0  UseKiTs=off  D=0.01  UseExternalDerivativeSource=off  N=10  UseFilter=on  TunerSelectOption=Transfer Function Based (PID Tuner App)  InitialConditionSource=internal  InitialConditionForIntegrator=0  InitialConditionForFilter=0  DifferentiatorICPrevScaledInput=0  ExternalReset=none  TrackingMode=off  Kt=1  LimitOutput=off  SatLimitsSource=internal  UpperSaturationLimit=inf  LowerSaturationLimit=-inf  LinearizeAsGain=on  AntiWindupMode=none  Kb=1  LimitIntegrator=off  UpperIntegratorSaturationLimit=inf  LowerIntegratorSaturationLimit=-inf  POutMin=[]  POutMax=[]  IOutMin=[]  IOutMax=[]  DOutMin=[]  DOutMax=[]  NOutMin=[]  NOutMax=[]  SumOutMin=[]  SumOutMax=[]  SaturationOutMin=[]  SaturationOutMax=[]  PParamMin=[]  PParamMax=[]  IParamMin=[]  IParamMax=[]  DParamMin=[]  DParamMax=[]  NParamMin=[]  NParamMax=[]  KbParamMin=[]  KbParamMax=[]  KtParamMin=[]  KtParamMax=[]  KbOutMin=[]  KbOutMax=[]  KtOutMin=[]  KtOutMax=[]  IntegratorOutMin=[]  IntegratorOutMax=[]  FilterOutMin=[]  FilterOutMax=[]  SumI1OutMin=[]  SumI1OutMax=[]  SumI2OutMin=[]  SumI2OutMax=[]  SumI3OutMin=[]  SumI3OutMax=[]  SumI4OutMin=[]  SumI4OutMax=[]  SumDOutMin=[]  SumDOutMax=[]  DifferentiatorOutMin=[]  DifferentiatorOutMax=[]  FilterDiffOutCoefMin=[]  FilterDiffOutCoefMax=[]  ReciprocalOutMin=[]  ReciprocalOutMax=[]  SumDenOutMin=[]  SumDenOutMax=[]  SumNumOutMin=[]  SumNumOutMax=[]  DivideOutMin=[]  DivideOutMax=[]  UdiffTsProdOutMin=[]  UdiffTsProdOutMax=[]  NTsProdOutMin=[]  NTsProdOutMax=[]  UintegralTsProdOutMin=[]  UintegralTsProdOutMax=[]  UngainTsProdOutMin=[]  UngainTsProdOutMax=[]  ClampingZeroOutDataTypeStr=Inherit: Inherit via back propagation  ClampingZeroOutMin=[]  ClampingZeroOutMax=[]  FilterDenConstantOutDataTypeStr=Inherit: Inherit via back propagation  FilterDenConstantOutMin=[]  FilterDenConstantOutMax=[]  PCopyOutDataTypeStr=Inherit: Inherit via back propagation  PCopyOutMin=[]  PCopyOutMax=[]  NCopyOutDataTypeStr=Inherit: Inherit via back propagation  NCopyOutMin=[]  NCopyOutMax=[]  IntegratorContinuousStateAttributes=''  IntegratorStateMustResolveToSignalObject=off  IntegratorRTWStateStorageClass=Auto  FilterContinuousStateAttributes=''  FilterStateMustResolveToSignalObject=off  FilterRTWStateStorageClass=Auto  ParallelPVariant=InternalParameters  IdealPVariant=Disabled  IVariant=InternalParameters  DVariant=InternalParameters  IntegratorVariant=Continuous  SatVariant=Disabled  AWVariant=Passthrough  PCopyVariant=Disabled  TRVariant=Disabled  FdbkBlocksVariant=Forward  IdealPFdbkVariant=Disabled  SatFdbkVariant=Disabled  DerivativeFilterVariant=ContFilter  NVariant=InternalParameters  NCopyVariant=Disabled  FilterICVariant=InternalICsFilter  IntegratorICVariant=InternalICs  ExternalResetVariant=Disabled  TRSumVariant=Passthrough  SumFdbkVariant=Disabled  SumVariant=Sum_PID  TsampFilterVariant=InternalTs  TsampNgainVariant=Passthrough  TsampIntegralVariant=Disabled_SignalSpec  ExternalSaturationOutDataTypeStr=Inherit: Same as second input  DerivativeSourceVariant=ErrorSignal  PreIntVariant=InternalPreInt
  Subsystem10 : Subsystem
  Subsystem11 : Subsystem
  Subsystem12 : Subsystem
  Subsystem13 : Subsystem
  Sum{28,30..32} (4 alike) : Sum  Inputs=|+-
  Transport Delay{9..12} (4 alike) : TransportDelay  DelayTime=120  InitialOutput=7
  Out1 : Outport
  Out2 : Outport  Port=2
  Out3 : Outport  Port=3
  Out4 : Outport  Port=4
  Out5 : Outport  Port=5
  Out6 : Outport  Port=6
  Out7 : Outport  Port=7
  Out8 : Outport  Port=8
  Out9 : Outport  Port=9
  Out10 : Outport  Port=10
  wires:
  Glucosa deseada13/1 -> Sum31/1
  Subsystem12/1(Out1) -> Out4/1, Insulina1/4, Insulina 2 min6/2
  2 min9/1 -> Out10/1, Glucosa1/5, Glucosa con Retardo 2min  y con PI7/2
  I.Basal6/1 -> Out1/1, Insulina1/1, Insulina 2 min4/1
  Transport Delay12/1 -> Sum32/2, 2 min9/1
  Glucosa deseada14/1 -> Sum32/1
  Gain31/1 -> Error10/1
  I.Basal9/1 -> Insulina 2 min7/1
  PID Controller13/1 -> Control12/1, Subsystem12/1(Controlador)
  Glucosa deseada11/1 -> Sum28/1
  I.Basal8/1 -> Insulina 2 min6/1
  Ingesta 75 g19/1(D) -> Subsystem13/2(D)
  Gb8/1 -> Glucosa con Retardo 2min  y con PI6/1
  2 min8/1 -> Out9/1, Glucosa1/4, Glucosa con Retardo 2min  y con PI6/2
  PID Controller12/1 -> Control11/1, Subsystem11/1(Controlador)
  Gb9/1 -> Glucosa con Retardo 2min  y con PI7/1
  Sum32/1 -> PID Controller14/1, Gain34/1
  Gb6/1 -> Out6/1, Glucosa1/1, Glucosa con Retardo 2min  y con PI4/1
  Transport Delay11/1 -> Sum31/2, 2 min8/1
  Clock18/1 -> Ingesta 75 g18/1(in)
  PID Controller14/1 -> Control13/1, Subsystem13/1(Controlador)
  Subsystem10/1(Out1) -> Insulina 2 min4/2, Out2/1, Insulina1/2
  PID Controller11/1 -> Control10/1, Subsystem10/1(Controlador)
  2 min6/1 -> Out7/1, Glucosa1/2, Glucosa con Retardo 2min  y con PI4/2
  Subsystem12/2(Out2) -> Transport Delay11/1
  Gb7/1 -> Glucosa con Retardo 2min  y con PI5/1
  Subsystem13/1(Out1) -> Out5/1, Insulina1/5, Insulina 2 min7/2
  Sum31/1 -> PID Controller13/1, Gain33/1
  2 min7/1 -> Out8/1, Glucosa1/3, Glucosa con Retardo 2min  y con PI5/2
  Subsystem13/2(Out2) -> Transport Delay12/1
  Gain33/1 -> Error12/1
  Transport Delay9/1 -> Sum28/2, 2 min6/1
  Constant25/1 -> Gb8/1
  Ingesta 75 g17/1(D) -> Subsystem11/2(D)
  Ingesta 75 g18/1(D) -> Subsystem12/2(D)
  Gain34/1 -> Error13/1
  Clock19/1 -> Ingesta 75 g19/1(in)
  Glucosa deseada12/1 -> Sum30/1
  Constant26/1 -> Gb9/1
  Ingesta 75 g16/1(D) -> Subsystem10/2(D)
  Subsystem11/1(Out1) -> Out3/1, Insulina1/3, Insulina 2 min5/2
  Sum28/1 -> PID Controller11/1, Gain31/1
  Constant23/1 -> Gb6/1
  Sum30/1 -> PID Controller12/1, Gain32/1
  Transport Delay10/1 -> Sum30/2, 2 min7/1
  I.Basal7/1 -> Insulina 2 min5/1
  Subsystem11/2(Out2) -> Transport Delay10/1
  Clock17/1 -> Ingesta 75 g17/1(in)
  Subsystem10/2(Out2) -> Transport Delay9/1
  Constant24/1 -> Gb7/1
  Gain32/1 -> Error11/1
  Clock16/1 -> Ingesta 75 g16/1(in)
